simulink model "soar_analysis_model"  (R2018b)
settings: Solver=ode4  StartTime=0.0  StopTime=60  FixedStep=simParams.sample_time_s  RelTol=1e-3
values from neighbouring files (symbols this model uses):
  hw_in = Aw * Jw * (RPM2RADPS * Om0)    [soar_analysis.m]
  omega_in = zeros(3,1) + var_w.*randn(3,1)    [soar_analysis.m]
  quat_in = [ cosd(ang/2); sind(ang/2).*ax ]    [soar_analysis.m]
undefined symbols (not defined in the file or in its folder): exitcode, final_time_s, fsw_telemetry_bus, fswParams, MET_epoch, omega_cmd, opt_ctrl_nm, opt_state, quat_cmd, quat_kinematics_lib, rigid_body_dynamics_lib, sc_mode, sI_unit, simParams, soar_count, soar_interface_lib, soarParams
libraries: simulink x4, quat_err_lib x1, quat_degerr_check x1, quat_degerr_lib x1, sharedutil x1, quat_rectify_lib x1, vrlib x1, aerolibutil x1, dspswit3 x1, soar_interp x1, soar_lib x1
settings Model: Creator=taylorreynolds  LastModifiedBy=Nick's PC
settings DebuggingCC: SingleTaskRateTransMsg=error
settings SFSimCC: SimUseLocalCustomCode=off
settings RTWCC: GenerateReport=on  RTWUseLocalCustomCode=off  LaunchReport=on
settings CodeAppCC: StateflowObjectComments=on

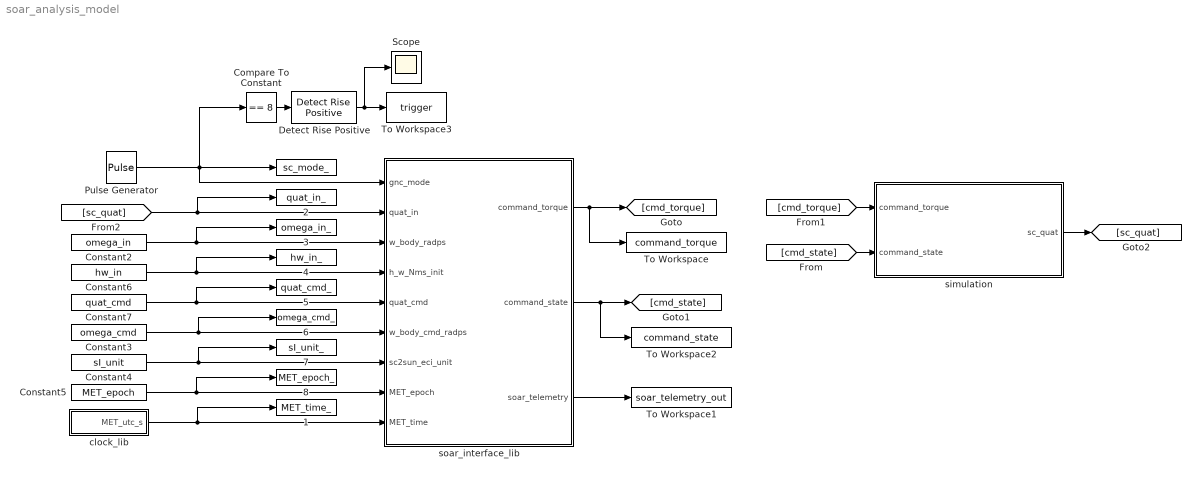
== system soar_analysis_model ==
  " " : ToWorkspace  VariableName=sc_mode_  SaveFormat=Timeseries  SampleTime=-1
  " 1" : ToWorkspace  VariableName=MET_time_  SaveFormat=Timeseries  SampleTime=-1
  " 2" : ToWorkspace  VariableName=quat_in_  SaveFormat=Timeseries  SampleTime=-1
  " 3" : ToWorkspace  VariableName=omega_in_  SaveFormat=Timeseries  SampleTime=-1
  " 4" : ToWorkspace  VariableName=hw_in_  SaveFormat=Timeseries  SampleTime=-1
  " 5" : ToWorkspace  VariableName=quat_cmd_  SaveFormat=Timeseries  SampleTime=-1
  " 6" : ToWorkspace  VariableName=omega_cmd_  SaveFormat=Timeseries  SampleTime=-1
  " 7" : ToWorkspace  VariableName=sI_unit_  SaveFormat=Timeseries  SampleTime=-1
  " 8" : ToWorkspace  VariableName=MET_epoch_  SaveFormat=Timeseries  SampleTime=-1
  Compare To Constant : simulink/Logic and Bit Operations/Compare To Constant  relop===  const=8  OutDataTypeStr=boolean
  Constant2 : Constant  Value=omega_in  SampleTime=-1
  Constant3 : Constant  Value=omega_cmd  SampleTime=-1
  Constant4 : Constant  Value=sI_unit  SampleTime=-1
  Constant5 : Constant  Value=MET_epoch  SampleTime=-1
  Constant6 : Constant  Value=hw_in  SampleTime=-1
  Constant7 : Constant  Value=quat_cmd  SampleTime=-1
  Detect Rise Positive : simulink/Logic and Bit Operations/Detect Rise Positive  vinit=0  OutDataTypeStr=boolean
  Pulse Generator : DiscretePulseGenerator  PulseType=Time based  Amplitude=sc_mode  Period=120  PulseWidth=5  SampleTime=simParams.sample_time_s
  Scope : Scope
  To Workspace : ToWorkspace  VariableName=command_torque  SampleTime=-1
  To Workspace1 : ToWorkspace  VariableName=soar_telemetry_out  SaveFormat=Timeseries  SampleTime=-1
  To Workspace2 : ToWorkspace  VariableName=command_state  SampleTime=-1
  To Workspace3 : ToWorkspace  VariableName=trigger  SampleTime=-1
  clock_lib : Subsystem
  simulation : Subsystem
  soar_interface_lib : Subsystem  AncestorBlock=soar_interface_lib/soar_interface_lib
  wires:
  Constant5/1 -> soar_interface_lib/8(MET_epoch), " 8"/1
  soar_interface_lib/1(command_torque) -> [cmd_torque], To Workspace/1
  soar_interface_lib/3(soar_telemetry) -> To Workspace1/1
  Constant6/1 -> soar_interface_lib/4(h_w_Nms_init), " 4"/1
  Constant7/1 -> soar_interface_lib/5(quat_cmd), " 5"/1
  Constant4/1 -> soar_interface_lib/7(sc2sun_eci_unit), " 7"/1
  Constant2/1 -> soar_interface_lib/3(w_body_radps), " 3"/1
  [sc_quat] -> soar_interface_lib/2(quat_in), " 2"/1
  soar_interface_lib/2(command_state) -> To Workspace2/1, [cmd_state]
  [cmd_torque] -> simulation/1(command_torque)
  [cmd_state] -> simulation/2("command_state ")
  Constant3/1 -> soar_interface_lib/6(w_body_cmd_radps), " 6"/1
  simulation/1(sc_quat) -> [sc_quat]
  Pulse Generator/1 -> soar_interface_lib/1(gnc_mode), Compare To Constant/1, " "/1
  Compare To Constant/1 -> Detect Rise Positive/1
  Detect Rise Positive/1 -> Scope/1, To Workspace3/1
  clock_lib/1(MET_utc_s) -> soar_interface_lib/9(MET_time), " 1"/1

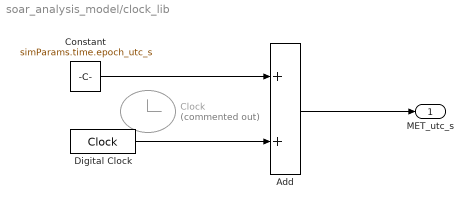
== system soar_analysis_model/clock_lib ==
  Add : Sum
  Clock : Clock  Commented=on
  Constant : Constant  Value=simParams.time.epoch_utc_s
  Digital Clock : DigitalClock  SampleTime=simParams.sample_time_s
  MET_utc_s : Outport
  wires:
  Digital Clock/1 -> Add/2
  Constant/1 -> Add/1
  Add/1 -> MET_utc_s/1

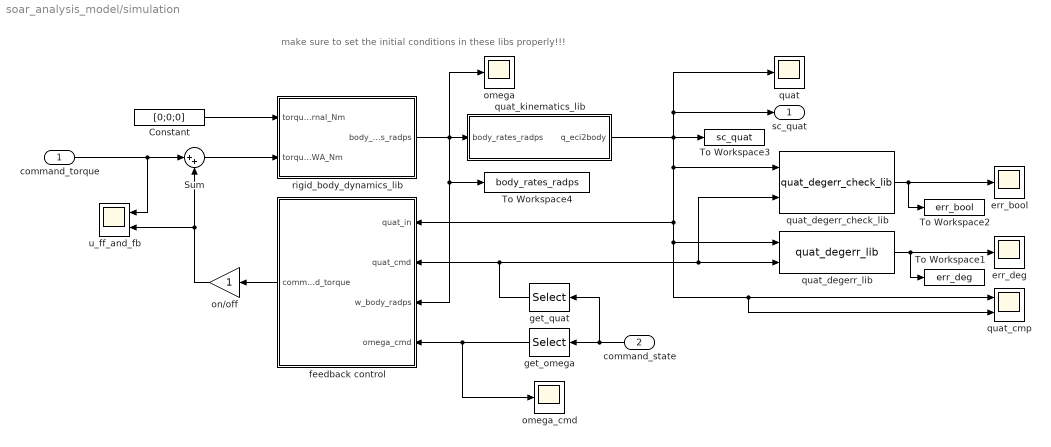
== system soar_analysis_model/simulation ==
  note: make sure to set the initial conditions in these libs properly!!!
  command_torque : Inport
  "command_state " : Inport  Port=2
  Constant : Constant  Value=[0;0;0]
  Sum : Sum  Inputs=|++
  To Workspace1 : ToWorkspace  VariableName=err_deg  SampleTime=-1
  To Workspace2 : ToWorkspace  VariableName=err_bool  SampleTime=-1
  To Workspace3 : ToWorkspace  VariableName=sc_quat  SampleTime=-1
  To Workspace4 : ToWorkspace  VariableName=body_rates_radps  SampleTime=-1
  err_bool : Scope
  err_deg : Scope
  feedback control : Subsystem
  get_omega : Selector  InputPortWidth=10  IndexOptions=Index vector (dialog)  Indices=[5 6 7]  OutputSizes=1
  get_quat : Selector  InputPortWidth=10  IndexOptions=Index vector (dialog)  Indices=[1 2 3 4]  OutputSizes=1
  omega : Scope
  omega_cmd : Scope
  on/off : Gain
  quat : Scope
  quat_cmp : Scope  NumInputPorts=2
  quat_degerr_check_lib : quat_degerr_check/quat_degerr_check_lib  point_tol=1
  quat_degerr_lib : quat_degerr_lib/quat_degerr_lib  SystemSampleTime=-1
  quat_kinematics_lib : Subsystem  AncestorBlock=quat_kinematics_lib/quat_kinematics_lib
  rigid_body_dynamics_lib : Subsystem  AncestorBlock=rigid_body_dynamics_lib/rigid_body_dynamics_lib
  u_ff_and_fb : Scope  NumInputPorts=2
  sc_quat : Outport
  wires:
  rigid_body_dynamics_lib/1(body_rates_radps) -> quat_kinematics_lib/1(body_rates_radps), feedback control/3(w_body_radps), To Workspace4/1, omega/1
  Constant/1 -> rigid_body_dynamics_lib/1(torque_external_Nm)
  quat_degerr_check_lib/1 -> To Workspace2/1, err_bool/1
  "command_state "/1 -> get_quat/1, get_omega/1
  Sum/1 -> rigid_body_dynamics_lib/2(torque_RWA_Nm)
  get_omega/1 -> omega_cmd/1, feedback control/4(omega_cmd)
  command_torque/1 -> u_ff_and_fb/1, Sum/1
  feedback control/1(command_torque) -> on/off/1
  on/off/1 -> u_ff_and_fb/2, Sum/2
  quat_degerr_lib/1 -> To Workspace1/1, err_deg/1
  quat_kinematics_lib/1(q_eci2body) -> sc_quat/1, quat/1, quat_degerr_lib/1, quat_cmp/2, quat_cmp/1, feedback control/1(quat_in), quat_degerr_check_lib/1, To Workspace3/1
  get_quat/1 -> quat_degerr_lib/2, quat_degerr_check_lib/2, feedback control/2(quat_cmd)

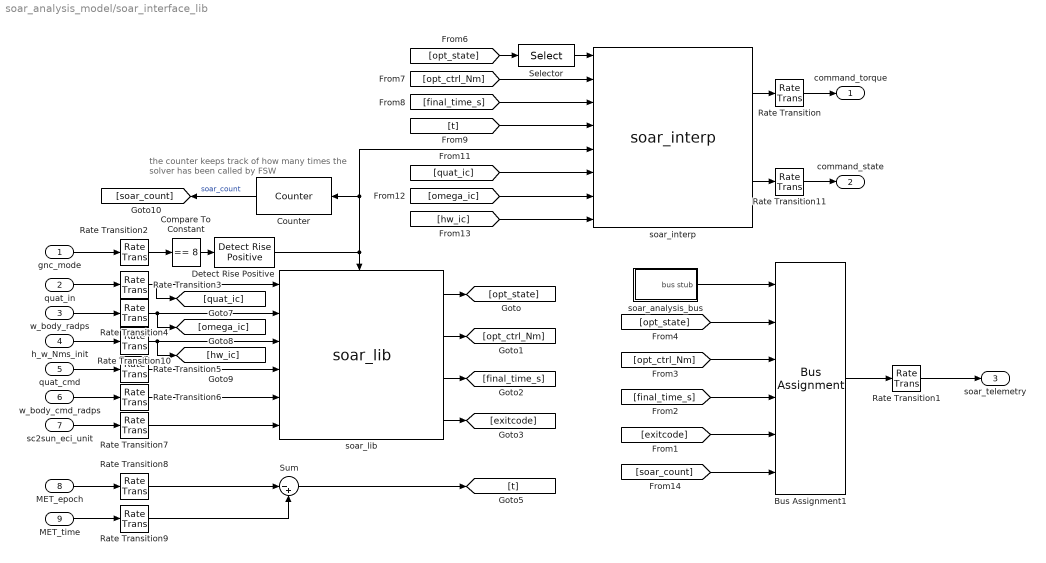
== system soar_analysis_model/soar_interface_lib ==
  note: the counter keeps track of how many times
      | the solver has been called by FSW
  gnc_mode : Inport
  quat_in : Inport  Port=2
  w_body_radps : Inport  Port=3
  h_w_Nms_init : Inport  Port=4
  quat_cmd : Inport  Port=5
  w_body_cmd_radps : Inport  Port=6
  sc2sun_eci_unit : Inport  Port=7
  MET_epoch : Inport  Port=8
  MET_time : Inport  Port=9
  Bus Assignment1 : BusAssignment  AssignedSignals=opt_state,opt_ctrl_nm,final_time_s,exitcode,soar_count
  Compare To Constant : simulink/Logic and Bit Operations/Compare To Constant  relop===  const=8  OutDataTypeStr=boolean
  Counter : dspswit3/Counter  Direction=Up  CountEvent=Rising edge  CounterSize=32 bits  MaxCount=255  InitialCount=0  Output=Count  HitValue=32  ResetInput=off  SamplesPerFrame=1  Ts=1  CntDtype=uint32  HitDtype=Logical
  Detect Rise Positive : simulink/Logic and Bit Operations/Detect Rise Positive  vinit=0  OutDataTypeStr=boolean
  Rate Transition : RateTransition
  Rate Transition1 : RateTransition  OutPortSampleTime=fswParams.sample_time_s
  Rate Transition{2,4,6..10} (7 alike) : RateTransition  OutPortSampleTime=soarParams.sample_time_s
  Rate Transition11 : RateTransition  InitialCondition=[quat_in; omega_in; hw_in]
  Rate Transition3 : RateTransition  InitialCondition=soarParams.ic.quat_in  OutPortSampleTime=soarParams.sample_time_s
  Rate Transition5 : RateTransition  InitialCondition=soarParams.ic.quat_cmd  OutPortSampleTime=soarParams.sample_time_s
  Selector : Selector  InputPortWidth=10*soarParams.N  IndexOptions=Index vector (dialog)  Indices=[91 92 93 94 95 96 97 98 99 100]  OutputSizes=1
  Sum : Sum  Inputs=|-+
  soar_analysis_bus : Subsystem  AncestorBlock=fsw_telemetry_bus/fsw_telemetry_bus
  soar_interp : soar_interp/soar_interp  SystemSampleTime=-1
  soar_lib : soar_lib/soar_lib  SystemSampleTime=-1
  command_torque : Outport
  command_state : Outport  Port=2
  soar_telemetry : Outport  Port=3  OutDataTypeStr=Bus: soar_telemetry
  wires:
  Selector/1 -> soar_interp/1
  soar_lib/3 -> [final_time_s]
  soar_lib/2 -> [opt_ctrl_Nm]
  h_w_Nms_init/1 -> Rate Transition10/1
  Rate Transition10/1 -> [hw_ic], soar_lib/3
  Rate Transition9/1 -> Sum/2
  Rate Transition8/1 -> Sum/1
  Rate Transition7/1 -> soar_lib/6
  Rate Transition6/1 -> soar_lib/5
  Rate Transition5/1 -> soar_lib/4
  Rate Transition4/1 -> [omega_ic], soar_lib/2
  Rate Transition3/1 -> soar_lib/1, [quat_ic]
  Rate Transition1/1 -> soar_telemetry/1
  [opt_state] -> Bus Assignment1/2
  [opt_ctrl_Nm] -> Bus Assignment1/3
  [final_time_s] -> Bus Assignment1/4
  [exitcode] -> Bus Assignment1/5
  Bus Assignment1/1 -> Rate Transition1/1
  Sum/1 -> [t]
  MET_time/1 -> Rate Transition9/1
  MET_epoch/1 -> Rate Transition8/1
  soar_lib/4 -> [exitcode]
  soar_lib/1 -> [opt_state]
  Compare To Constant/1 -> Detect Rise Positive/1
  gnc_mode/1 -> Rate Transition2/1
  sc2sun_eci_unit/1 -> Rate Transition7/1
  w_body_cmd_radps/1 -> Rate Transition6/1
  quat_cmd/1 -> Rate Transition5/1
  w_body_radps/1 -> Rate Transition4/1
  quat_in/1 -> Rate Transition3/1
  Rate Transition2/1 -> Compare To Constant/1
  soar_interp/1 -> Rate Transition/1
  soar_interp/2 -> Rate Transition11/1
  Counter/1 -> [soar_count]  "soar_count"
  [opt_state] -> Selector/1
  [opt_ctrl_Nm] -> soar_interp/2
  [final_time_s] -> soar_interp/3
  [t] -> soar_interp/4
  Detect Rise Positive/1 -> Counter/1, soar_interp/5, soar_lib/Trigger
  [quat_ic] -> soar_interp/6
  [omega_ic] -> soar_interp/7
  [hw_ic] -> soar_interp/8
  Rate Transition/1 -> command_torque/1
  Rate Transition11/1 -> command_state/1
  [soar_count] -> Bus Assignment1/6
  soar_analysis_bus/1(bus stub) -> Bus Assignment1/1

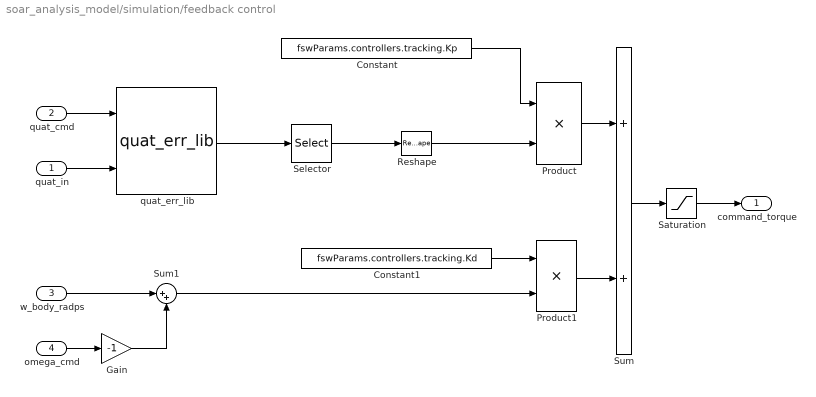
== system soar_analysis_model/simulation/feedback control ==
  quat_in : Inport
  quat_cmd : Inport  Port=2
  w_body_radps : Inport  Port=3
  omega_cmd : Inport  Port=4
  Constant : Constant  Value=fswParams.controllers.tracking.Kp
  Constant1 : Constant  Value=fswParams.controllers.tracking.Kd
  Gain : Gain  Gain=-1
  Product : Product
  Product1 : Product
  Reshape : Reshape
  Saturation : Saturate  UpperLimit=simParams.actuators.rwa.max_torque_Nm  LowerLimit=-simParams.actuators.rwa.max_torque_Nm
  Selector : Selector  InputPortWidth=4  IndexOptions=Index vector (dialog)  Indices=[2 3 4]  OutputSizes=1
  Sum : Sum
  Sum1 : Sum  Inputs=|++
  quat_err_lib : quat_err_lib/quat_err_lib  SystemSampleTime=-1
  command_torque : Outport
  wires:
  Selector/1 -> Reshape/1
  Sum1/1 -> Product1/2
  Gain/1 -> Sum1/2
  omega_cmd/1 -> Gain/1
  w_body_radps/1 -> Sum1/1
  Saturation/1 -> command_torque/1
  Product1/1 -> Sum/2
  Product/1 -> Sum/1
  Constant/1 -> Product/1
  Constant1/1 -> Product1/1
  Sum/1 -> Saturation/1
  quat_cmd/1 -> quat_err_lib/1
  quat_in/1 -> quat_err_lib/2
  quat_err_lib/1 -> Selector/1
  Reshape/1 -> Product/2

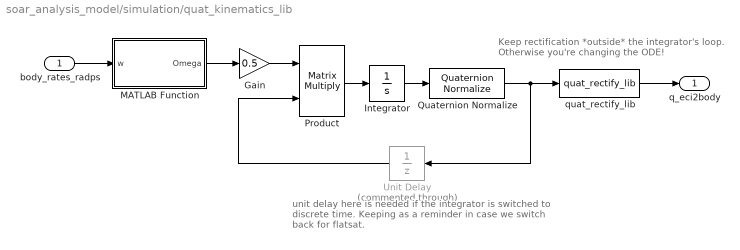
== system soar_analysis_model/simulation/quat_kinematics_lib ==
  note: unit delay here is needed if the integrator is
      | switched to discrete time. Keeping as a reminder
      | in case we switch back for flatsat.
  note: Keep rectification *outside* the integrator's
      | loop. Otherwise you're changing the ODE!
  body_rates_radps : Inport
  Gain : Gain  Gain=0.5
  Integrator : Integrator  InitialCondition=quat_in
  MATLAB Function : MATLAB Function  TreatAsAtomicUnit=on
  Product : Product  Multiplication=Matrix(*)
  Quaternion Normalize : sharedutil/Quaternion Normalize  aMode=aMode
      settings: SourceProductName=Aerospace Blockset  SourceProductBaseCode=AE
  Unit Delay : UnitDelay  Commented=through  InitialCondition=simParams.initialConditions.q_eci2body  SampleTime=-1
  quat_rectify_lib : quat_rectify_lib/quat_rectify_lib
  q_eci2body : Outport
  wires:
  quat_rectify_lib/1 -> q_eci2body/1
  Quaternion Normalize/1 -> quat_rectify_lib/1, Unit Delay/1
  Unit Delay/1 -> Product/2
  Gain/1 -> Product/1
  Product/1 -> Integrator/1
  MATLAB Function/1(Omega) -> Gain/1
  body_rates_radps/1 -> MATLAB Function/1(w)
  Integrator/1 -> Quaternion Normalize/1

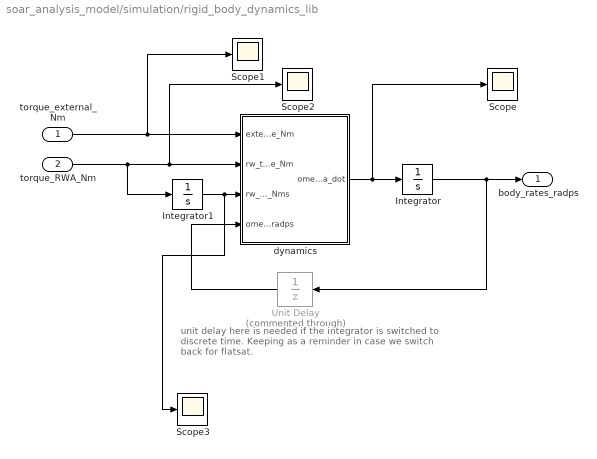
== system soar_analysis_model/simulation/rigid_body_dynamics_lib ==
  note: unit delay here is needed if the integrator is
      | switched to discrete time. Keeping as a reminder
      | in case we switch back for flatsat.
  torque_external_Nm : Inport
  torque_RWA_Nm : Inport  Port=2
  Integrator : Integrator  InitialCondition=omega_in
  Integrator1 : Integrator  InitialCondition=hw_in
  Scope{,1..3} (4 alike) : Scope
  Unit Delay : UnitDelay  Commented=through  InitialCondition=simParams.initialConditions.w_body_radps  SampleTime=-1
  dynamics : Subsystem
  body_rates_radps : Outport
  wires:
  Unit Delay/1 -> dynamics/4(omega_radps)
  dynamics/1(omega_dot) -> Scope/1, Integrator/1
  Integrator1/1 -> Scope3/1, dynamics/3(rw_momentum_Nms)
  Integrator/1 -> body_rates_radps/1, Unit Delay/1
  torque_external_Nm/1 -> Scope1/1, dynamics/1(external_torque_Nm)
  torque_RWA_Nm/1 -> Scope2/1, dynamics/2(rw_torque_Nm), Integrator1/1

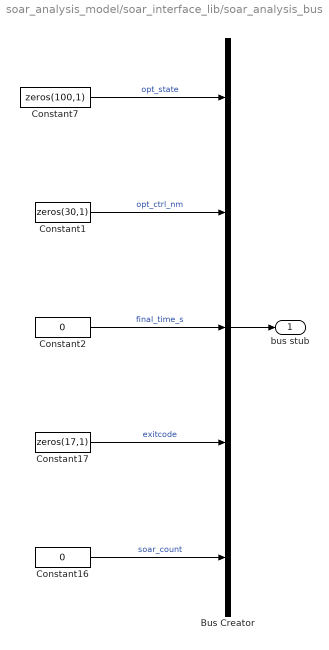
== system soar_analysis_model/soar_interface_lib/soar_analysis_bus ==
  Bus Creator : BusCreator  Inputs=5
  Constant1 : Constant  Value=zeros(30,1)  OutDataTypeStr=double  SampleTime=fswParams.sample_time_s
  Constant16 : Constant  Value=0  OutDataTypeStr=uint32  SampleTime=fswParams.sample_time_s
  Constant17 : Constant  Value=zeros(17,1)  OutDataTypeStr=double  SampleTime=fswParams.sample_time_s
  Constant2 : Constant  Value=0  OutDataTypeStr=double  SampleTime=fswParams.sample_time_s
  Constant7 : Constant  Value=zeros(100,1)  OutDataTypeStr=double  SampleTime=fswParams.sample_time_s
  bus stub : Outport
  wires:
  Constant17/1 -> Bus Creator/4  "exitcode"
  Constant16/1 -> Bus Creator/5  "soar_count"
  Constant2/1 -> Bus Creator/3  "final_time_s"
  Constant1/1 -> Bus Creator/2  "opt_ctrl_nm"
  Constant7/1 -> Bus Creator/1  "opt_state"
  Bus Creator/1 -> bus stub/1

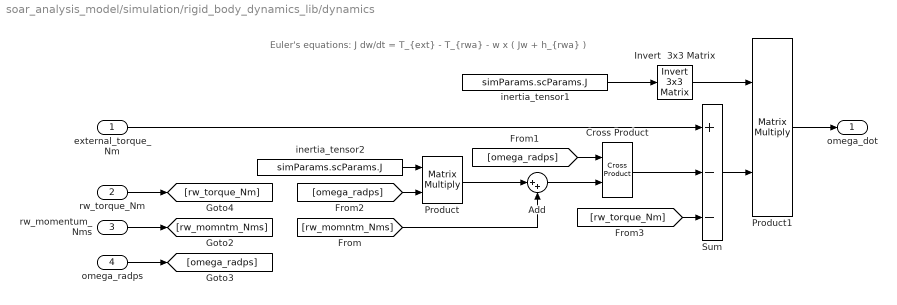
== system soar_analysis_model/simulation/rigid_body_dynamics_lib/dynamics ==
  note: Euler's equations: J dw/dt = T_{ext} - T_{rwa} - w x ( Jw + h_{rwa} )
  external_torque_Nm : Inport
  rw_torque_Nm : Inport  Port=2
  rw_momentum_Nms : Inport  Port=3
  omega_radps : Inport  Port=4
  Add : Sum  Inputs=|++
  Cross Product : vrlib/Utilities/Cross Product
      settings: SourceProductBaseCode=VR
  Invert  3x3 Matrix : aerolibutil/Invert  3x3 Matrix
  Product : Product  Multiplication=Matrix(*)  RndMeth=Zero
  Product1 : Product  Multiplication=Matrix(*)  RndMeth=Zero
  Sum : Sum  Inputs=+--
  inertia_tensor1 : Constant  Value=simParams.scParams.J  SampleTime=simParams.sample_time_s
  inertia_tensor2 : Constant  Value=simParams.scParams.J  SampleTime=simParams.sample_time_s
  omega_dot : Outport
  wires:
  [rw_torque_Nm] -> Sum/3
  [omega_radps] -> Product/2
  [omega_radps] -> Cross Product/1
  [rw_momntm_Nms] -> Add/2
  rw_momentum_Nms/1 -> [rw_momntm_Nms]
  external_torque_Nm/1 -> Sum/1
  omega_radps/1 -> [omega_radps]
  inertia_tensor2/1 -> Product/1
  Sum/1 -> Product1/2
  Product1/1 -> omega_dot/1
  Invert  3x3 Matrix/1 -> Product1/1
  inertia_tensor1/1 -> Invert  3x3 Matrix/1
  Cross Product/1 -> Sum/2
  Product/1 -> Add/1
  Add/1 -> Cross Product/2
  rw_torque_Nm/1 -> [rw_torque_Nm]

== matlab function soar_analysis_model/simulation/quat_kinematics_lib/MATLAB Function ==
  data: w input; Omega output
function Omega = q_skew_star(w)
%#codegen
Omega = [ 0.0,  -w(1), -w(2), -w(3);
          w(1),  0.0,   w(3), -w(2);
          w(2), -w(3),  0.0,   w(1);
          w(3),  w(2), -w(1),  0.0 ];
end
